simulink model "projectmodel"  (R2016a)
settings: Solver=ode23tb  StartTime=0.0  StopTime=20  MaxStep=1e-3  RelTol=1e-3
values from neighbouring files (symbols this model uses):
  Supply_pr_Ps = 2.1e7    (= 21000000)    [data4_mfile.m]    (also in data8_mfile.m)
  Valve_eta = 0.989    [data4_mfile.m]    (also in data8_mfile.m = 0.99)
  Valve_omega = 40.5    [data4_mfile.m]    (also in data8_mfile.m = 38)
undefined symbols (not defined in the file or in its folder): Arm, Boom, Bucket, Cyl, Hose, Valve
libraries: mblibv1 x13, simulink x3, vrlib x2
settings Model: Creator=bangalor  LastModifiedBy=bangalor

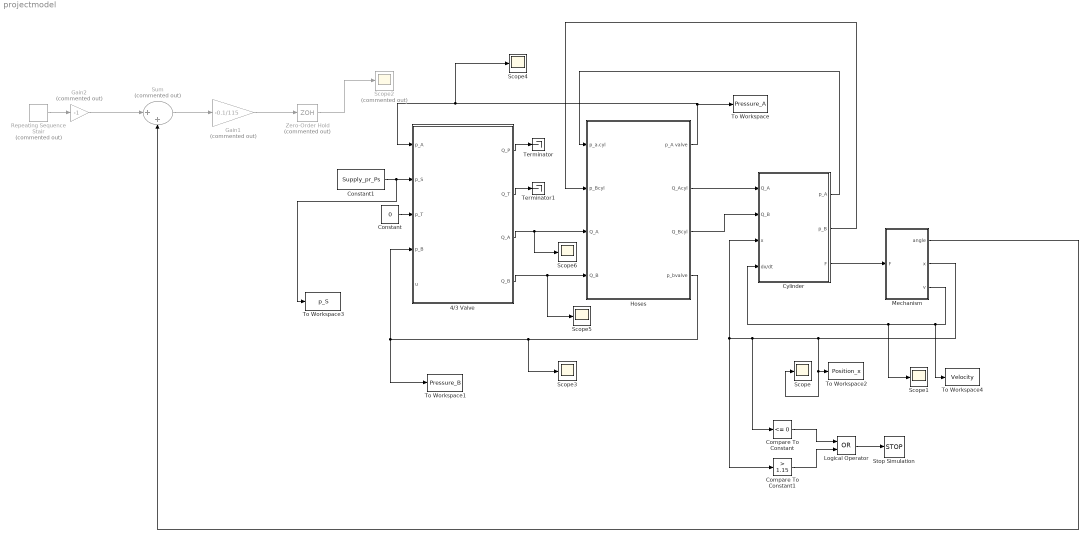
== system projectmodel ==
  4/3 Valve : Subsystem
  Compare To Constant : simulink/Logic and Bit Operations/Compare To Constant  relop=<=  const=0  OutDataTypeStr=boolean
  Compare To Constant1 : simulink/Logic and Bit Operations/Compare To Constant  relop=>  const=1.15  OutDataTypeStr=boolean
  Constant : Constant  Value=0
  Constant1 : Constant  Value=Supply_pr_Ps
  Cylinder : Subsystem
  Gain1 : Gain  Commented=on  Gain=-0.1/115
  Gain2 : Gain  Commented=on  Gain=-1
  Hoses : Subsystem
  Logical Operator : Logic  Operator=OR  AllPortsSameDT=off  OutDataTypeStr=boolean
  Mechanism : Subsystem
  Repeating Sequence Stair : simulink/Sources/Repeating Sequence Stair  Commented=on  OutValues=[50 72 94 115].'  tsamp=5  OutMin=[]  OutMax=[]  OutDataTypeStr=double  OutputDataTypeScalingMode=double  OutDataType=fixdt(0,8)  ConRadixGroup=Best Precision: Vector-wise  OutScaling=2^-12
  Scope{,1,3..6} (6 alike) : Scope
  Scope2 : Scope  Commented=on
  Stop Simulation : Stop
  Sum : Sum  Commented=on  Inputs=|++
  Terminator : Terminator
  Terminator1 : Terminator
  To Workspace : ToWorkspace  VariableName=Pressure_A  SampleTime=-1
  To Workspace1 : ToWorkspace  VariableName=Pressure_B  SampleTime=-1
  To Workspace2 : ToWorkspace  VariableName=Position_x  SampleTime=-1
  To Workspace3 : ToWorkspace  VariableName=p_S  SampleTime=-1
  To Workspace4 : ToWorkspace  VariableName=Velocity  SampleTime=-1
  Zero-Order Hold : ZeroOrderHold  Commented=on  SampleTime=50e-3
  wires:
  4/3 Valve/3(Q_A) -> Scope6/1, Hoses/3(Q_A)
  4/3 Valve/4(Q_B) -> Scope5/1, Hoses/4(Q_B)
  Mechanism/3(v) -> Cylinder/4(dx/dt), Scope1/1, To Workspace4/1
  Hoses/4(p_bvalve) -> Scope3/1, To Workspace1/1, 4/3 Valve/4(p_B)
  Hoses/1(p_A valve) -> Scope4/1, 4/3 Valve/1(p_A), To Workspace/1
  Hoses/2(Q_Acyl) -> Cylinder/1(Q_A)
  Hoses/3(Q_Bcyl) -> Cylinder/2(Q_B)
  Cylinder/1(p_A) -> Hoses/1(p_a.cyl)
  Cylinder/2(p_B) -> Hoses/2(p_Bcyl)
  4/3 Valve/1(Q_P) -> Terminator/1
  4/3 Valve/2(Q_T) -> Terminator1/1
  Constant/1 -> 4/3 Valve/3(p_T)
  Constant1/1 -> To Workspace3/1, 4/3 Valve/2(p_S)
  Cylinder/3(F) -> Mechanism/1(F)
  Sum/1 -> Gain1/1
  Gain1/1 -> Zero-Order Hold/1
  Mechanism/1(angle) -> Sum/2
  Repeating Sequence Stair/1 -> Gain2/1
  Zero-Order Hold/1 -> Scope2/1
  Gain2/1 -> Sum/1
  Mechanism/2(x) -> Scope/1, To Workspace2/1, Compare To Constant/1, Compare To Constant1/1, Cylinder/3(x)
  Compare To Constant/1 -> Logical Operator/1
  Compare To Constant1/1 -> Logical Operator/2
  Logical Operator/1 -> Stop Simulation/1

== system projectmodel/4//3 Valve ==
  p_A : Inport
  p_S : Inport  Port=2
  p_T : Inport  Port=3
  p_B : Inport  Port=4
  u : Inport  Port=5
  Flow paths : Subsystem
  From Workspace : FromWorkspace  VariableName=U_signal  SampleTime=1.0000e-03
  Relative openings : Subsystem
  Scope6 : Scope
  Valve Dynamics : Subsystem
  Q_P : Outport
  Q_T : Outport  Port=2
  Q_A : Outport  Port=3
  Q_B : Outport  Port=4
  wires:
  Valve Dynamics/1(x) -> Scope6/1, Relative openings/1(x)
  Relative openings/1(av_AT) -> Flow paths/5(av_AT)
  Flow paths/4(Q_B) -> Q_B/1
  Flow paths/3(Q_T) -> Q_T/1
  Flow paths/2(Q_P) -> Q_P/1
  Flow paths/1(Q_A) -> Q_A/1
  p_T/1 -> Flow paths/4(p_T)
  p_S/1 -> Flow paths/3(p_S)
  p_B/1 -> Flow paths/2(p_B)
  p_A/1 -> Flow paths/1(p_A)
  Relative openings/2(av_BT) -> Flow paths/6(av_BT)
  Relative openings/3(av_PB) -> Flow paths/7(av_PB)
  Relative openings/4(av_PA) -> Flow paths/8(av_PA)
  From Workspace/1 -> Valve Dynamics/1(u)

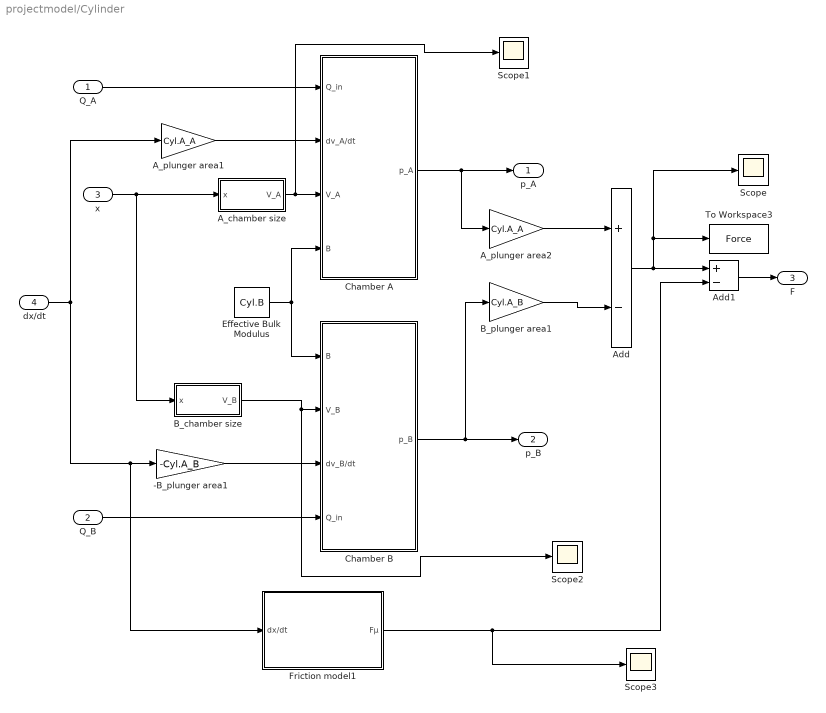
== system projectmodel/Cylinder ==
  Q_A : Inport
  Q_B : Inport  Port=2
  x : Inport  Port=3
  dx/dt : Inport  Port=4
  -B_plunger area1 : Gain  Gain=-Cyl.A_B
  A_chamber size : Subsystem
  A_plunger area1 : Gain  Gain=Cyl.A_A
  A_plunger area2 : Gain  Gain=Cyl.A_A
  Add : Sum  Inputs=+-
  Add1 : Sum  Inputs=+-
  B_chamber size : Subsystem
  B_plunger area1 : Gain  Gain=Cyl.A_B
  Chamber A : Subsystem  mask(Hydraulic){pinitial=Cyl.pa_init}
      mask prompts: pinitial "Initial pressure [Pa] :"
      mask help: Lumped fluid volume. Pressure is limited greater or equal to zero by saturation block corresponding to a rough model of cavitation.
      mask Help: eval('hydlibdoc(''vol_cav_doc'')')
  Chamber B : Subsystem  mask(Hydraulic){pinitial=Cyl.pb_init}
      mask prompts: pinitial "Initial pressure [Pa] :"
      mask help: Lumped fluid volume. Pressure is limited greater or equal to zero by saturation block corresponding to a rough model of cavitation.
      mask Help: eval('hydlibdoc(''vol_cav_doc'')')
  Effective Bulk Modulus : Constant  Value=Cyl.B
  Friction model1 : Subsystem
  Scope{,1..3} (4 alike) : Scope
  To Workspace3 : ToWorkspace  VariableName=Force  SampleTime=-1
  p_A : Outport
  p_B : Outport  Port=2
  F : Outport  Port=3
  wires:
  A_plunger area1/1 -> Chamber A/2(" dv_A/dt")
  dx/dt/1 -> A_plunger area1/1, Friction model1/1(dx/dt), -B_plunger area1/1
  Effective Bulk Modulus/1 -> Chamber A/4(" B"), Chamber B/1(B)
  x/1 -> B_chamber size/1(x), A_chamber size/1(x)
  -B_plunger area1/1 -> Chamber B/3(dv_B/dt)
  A_chamber size/1(V_A) -> Scope1/1, Chamber A/3(" V_A")
  Friction model1/1(Fµ) -> Add1/2, Scope3/1
  Q_A/1 -> Chamber A/1(Q_in)
  Chamber A/1(p_A) -> p_A/1, A_plunger area2/1
  Chamber B/1(p_B) -> p_B/1, B_plunger area1/1
  A_plunger area2/1 -> Add/1
  B_plunger area1/1 -> Add/2
  Add/1 -> Add1/1, To Workspace3/1, Scope/1
  B_chamber size/1(V_B) -> Scope2/1, Chamber B/2(V_B)
  Q_B/1 -> Chamber B/4(Q_in)
  Add1/1 -> F/1

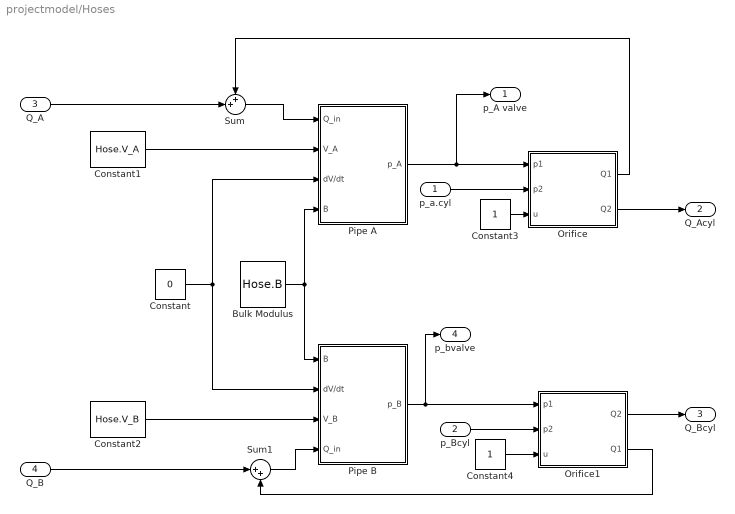
== system projectmodel/Hoses ==
  p_a.cyl : Inport
  p_Bcyl : Inport  Port=2
  Q_A : Inport  Port=3
  Q_B : Inport  Port=4
  Bulk Modulus : Constant  Value=Hose.B
  Constant : Constant  Value=0
  Constant1 : Constant  Value=Hose.V_A
  Constant2 : Constant  Value=Hose.V_B
  Constant3 : Constant
  Constant4 : Constant
  Orifice : Subsystem  mask(Hydraulic){QN=Hose.QN, dpN=Hose.dpN, ptr=Hose.ptr}
      mask prompts: QN "Nominal Flow [m^3/s] :"; dpN "Nominal Pressure Difference [Pa] :"; ptr "Transition Pressure [Pa] :"
      mask help:
      | Implements numerically robust turbulent flow
      | equation. Polynomial flow equation is used
      | when abs(dp) < Transition Pressure.
      mask init:
      | K = QN/(sqrt(dpN));
      mask Help: eval('hydlibdoc(''orificedoc'')')
  Orifice1 : Subsystem  mask(Hydraulic){QN=Hose.QN, dpN=Hose.dpN, ptr=Hose.ptr}
      mask prompts: QN "Nominal Flow [m^3/s] :"; dpN "Nominal Pressure Difference [Pa] :"; ptr "Transition Pressure [Pa] :"
      mask help:
      | Implements numerically robust turbulent flow
      | equation. Polynomial flow equation is used
      | when abs(dp) < Transition Pressure.
      mask init:
      | K = QN/(sqrt(dpN));
      mask Help: eval('hydlibdoc(''orificedoc'')')
  Pipe A : Subsystem  mask(Hydraulic){pinitial=Hose.pa_init}
      mask prompts: pinitial "Initial pressure [Pa] :"
      mask help: Lumped fluid volume. Pressure is limited greater or equal to zero by saturation block corresponding to a rough model of cavitation.
      mask Help: eval('hydlibdoc(''vol_cav_doc'')')
  Pipe B : Subsystem  mask(Hydraulic){pinitial=Hose.pb_init}
      mask prompts: pinitial "Initial pressure [Pa] :"
      mask help: Lumped fluid volume. Pressure is limited greater or equal to zero by saturation block corresponding to a rough model of cavitation.
      mask Help: eval('hydlibdoc(''vol_cav_doc'')')
  Sum : Sum  Inputs=++|
  Sum1 : Sum  Inputs=|++
  p_A valve : Outport
  Q_Acyl : Outport  Port=2
  Q_Bcyl : Outport  Port=3
  p_bvalve : Outport  Port=4
  wires:
  Q_B/1 -> Sum1/1
  Constant4/1 -> Orifice1/3(u)
  Constant2/1 -> Pipe B/3(V_B)
  Pipe A/1(p_A) -> p_A valve/1, Orifice/1(p1)
  p_a.cyl/1 -> Orifice/2(p2)
  Orifice/1(Q1) -> Sum/1
  Orifice/2(Q2) -> Q_Acyl/1
  Q_A/1 -> Sum/2
  Sum/1 -> Pipe A/1(Q_in)
  Pipe B/1(p_B) -> p_bvalve/1, Orifice1/1(p1)
  Orifice1/2(Q1) -> Sum1/2
  Sum1/1 -> Pipe B/4(" Q_in")
  Orifice1/1(Q2) -> Q_Bcyl/1
  Bulk Modulus/1 -> Pipe A/4(" B"), Pipe B/1(B)
  Constant/1 -> Pipe A/3(" dV/dt"), Pipe B/2(" dV/dt")
  Constant1/1 -> Pipe A/2(" V_A")
  Constant3/1 -> Orifice/3(u)
  p_Bcyl/1 -> Orifice1/2(p2)

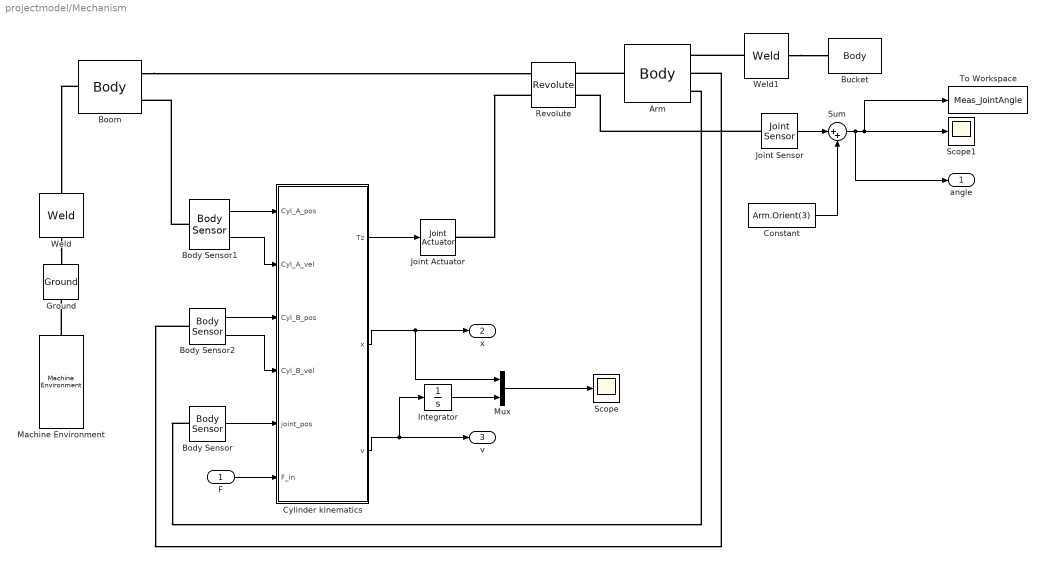
== system projectmodel/Mechanism ==
  F : Inport
  Arm : mblibv1/Bodies/Body  LConnTagsString=CS1  RConnTagsString=CS3|CS2|CS4  UpdateFromCAD=off  DialogClass=MechanicalBodyBlock  Mass=Arm.Mass  MassUnits=kg  InertiaUnits=kg*m^2  Inertia=Arm.Inertia  Shape=Cylinder  ShapeDims=[1 1]  ShapeUnits=m  ShapeUse=false  Density=1  DensityUnits=kg/m^3  DensityUse=false  GraphicsMode=MACHINE_DEFAULT  BodyColorSelMode=MACHINE_DEFAULT  BodyColor=[1 0 0]  AttachedToCS=CG  CG=Left$CG$Arm.CG$CS1$CS1$m$[0 0 0]$Euler X-Y-Z$deg$CS1$false$none  WorkingFrames=Left$CS1$[0 0 0]$Adjoining$Adjoining$m$Arm.Orient$Euler X-Y-Z$deg$Adjoining$true$none#Right$CS3$Arm.BucketJoint$CS1$CS1$m$[0 0 0]$Euler X-Y-Z$deg$CS1$true$none#Right$CS2$Arm.CylJoint$CS1$CS1$m$[0 0 0]$Euler X-Y-Z$deg$CS1$true$none#Right$CS4$[0 0 0]$CS1$CS1$m$[0 0 0]$Euler X-Y-Z$deg$CS1$true$none  CGPos=Arm.CG  CGRot=[0 0 0]  CS0Pos=[]  CS0Rot=[]  CS1Pos=[0 0 0]  CS1Rot=Arm.Orient  CS2Pos=Arm.CylJoint  CS2Rot=[0 0 0]  CS3Pos=Arm.BucketJoint  CS3Rot=[0 0 0]  CS4Pos=[0 0 0]  CS4Rot=[0 0 0]  CS5Pos=[]  CS5Rot=[]  CS6Pos=[]  CS6Rot=[]  CS7Pos=[]  CS7Rot=[]  CS8Pos=[]  CS8Rot=[]  CS9Pos=[]  CS9Rot=[]  CS10Pos=[]  CS10Rot=[]  CS11Pos=[]  CS11Rot=[]  CS12Pos=[]  CS12Rot=[]  CS13Pos=[]  CS13Rot=[]  CS14Pos=[]  CS14Rot=[]  CS15Pos=[]  CS15Rot=[]  CS16Pos=[]  CS16Rot=[]  CS17Pos=[]  CS17Rot=[]  CS18Pos=[]  CS18Rot=[]  CS19Pos=[]  CS19Rot=[]  CS20Pos=[]  CS20Rot=[]
  Body Sensor : mblibv1/Sensors &  Actuators/Body Sensor  UpdateFromCAD=off  PhysicalDomain=Mechanical  PortType=blob  Muxed=off  Pose=off  Angle=on  AngleUnits=deg  ArcVelocity=off  ArcVelocityUnits=deg/s  ArcAcceleration=off  ArcAccelerationUnits=deg/s^2  CoordPosition=on  CoordPositionUnits=m  Velocity=off  VelocityUnits=m/s  Acceleration=off  AccelerationUnits=m/s^2  Quaternion=on  QuaternionDT=off  QuaternionDDT=off  QuaternionUnits=off  OutputVector=[1]  ActiveIO=on  Width=3  DialogClass=MechanicalSensorBlock  ReferenceFrame=Absolute (World)
  Body Sensor1 : mblibv1/Sensors &  Actuators/Body Sensor  UpdateFromCAD=off  PhysicalDomain=Mechanical  PortType=blob  Muxed=off  Pose=off  Angle=on  AngleUnits=deg  ArcVelocity=off  ArcVelocityUnits=deg/s  ArcAcceleration=off  ArcAccelerationUnits=deg/s^2  CoordPosition=on  CoordPositionUnits=m  Velocity=on  VelocityUnits=m/s  Acceleration=off  AccelerationUnits=m/s^2  Quaternion=on  QuaternionDT=off  QuaternionDDT=off  QuaternionUnits=off  OutputVector=[1]  ActiveIO=on  Width=6  DialogClass=MechanicalSensorBlock  ReferenceFrame=Absolute (World)
  Body Sensor2 : mblibv1/Sensors &  Actuators/Body Sensor  UpdateFromCAD=off  PhysicalDomain=Mechanical  PortType=blob  Muxed=off  Pose=off  Angle=on  AngleUnits=deg  ArcVelocity=off  ArcVelocityUnits=deg/s  ArcAcceleration=off  ArcAccelerationUnits=deg/s^2  CoordPosition=on  CoordPositionUnits=m  Velocity=on  VelocityUnits=m/s  Acceleration=off  AccelerationUnits=m/s^2  Quaternion=on  QuaternionDT=off  QuaternionDDT=off  QuaternionUnits=off  OutputVector=[1]  ActiveIO=on  Width=6  DialogClass=MechanicalSensorBlock  ReferenceFrame=Absolute (World)
  Boom : mblibv1/Bodies/Body  LConnTagsString=CS1  RConnTagsString=CS2|CS3  UpdateFromCAD=off  DialogClass=MechanicalBodyBlock  Mass=Boom.Mass  MassUnits=kg  InertiaUnits=kg*m^2  Inertia=Boom.Inert  Shape=Cylinder  ShapeDims=[1 1]  ShapeUnits=m  ShapeUse=false  Density=1  DensityUnits=kg/m^3  DensityUse=false  GraphicsMode=MACHINE_DEFAULT  BodyColorSelMode=MACHINE_DEFAULT  BodyColor=[1 0 0]  AttachedToCS=CG  CG=Left$CG$[0 0 0]$CS1$CS1$m$[0 0 0]$Euler X-Y-Z$deg$CS1$false$none  WorkingFrames=Left$CS1$[0 0 0]$Adjoining$Adjoining$m$[0 0 0]$Euler X-Y-Z$deg$Adjoining$true$none#Right$CS2$Boom.ArmJoint$CS1$CS1$m$[0 0 0]$Euler X-Y-Z$deg$CS1$true$none#Right$CS3$Boom.CylJoint$CS1$CS1$m$[0 0 0]$Euler X-Y-Z$deg$CS1$true$none  CGPos=[0 0 0]  CGRot=[0 0 0]  CS0Pos=[]  CS0Rot=[]  CS1Pos=[0 0 0]  CS1Rot=[0 0 0]  CS2Pos=Boom.ArmJoint  CS2Rot=[0 0 0]  CS3Pos=Boom.CylJoint  CS3Rot=[0 0 0]  CS4Pos=[]  CS4Rot=[]  CS5Pos=[]  CS5Rot=[]  CS6Pos=[]  CS6Rot=[]  CS7Pos=[]  CS7Rot=[]  CS8Pos=[]  CS8Rot=[]  CS9Pos=[]  CS9Rot=[]  CS10Pos=[]  CS10Rot=[]  CS11Pos=[]  CS11Rot=[]  CS12Pos=[]  CS12Rot=[]  CS13Pos=[]  CS13Rot=[]  CS14Pos=[]  CS14Rot=[]  CS15Pos=[]  CS15Rot=[]  CS16Pos=[]  CS16Rot=[]  CS17Pos=[]  CS17Rot=[]  CS18Pos=[]  CS18Rot=[]  CS19Pos=[]  CS19Rot=[]  CS20Pos=[]  CS20Rot=[]
  Bucket : mblibv1/Bodies/Body  LConnTagsString=CS1  UpdateFromCAD=off  DialogClass=MechanicalBodyBlock  Mass=Bucket.Mass  MassUnits=kg  InertiaUnits=kg*m^2  Inertia=Bucket.Interia  Shape=Cylinder  ShapeDims=[1 1]  ShapeUnits=m  ShapeUse=false  Density=1  DensityUnits=kg/m^3  DensityUse=false  GraphicsMode=MACHINE_DEFAULT  BodyColorSelMode=MACHINE_DEFAULT  BodyColor=[1 0 0]  AttachedToCS=CG  CG=Left$CG$Bucket.CG$CS1$CS1$m$[0 0 0]$Euler X-Y-Z$deg$CS1$false$none  WorkingFrames=Left$CS1$[0 0 0]$Adjoining$Adjoining$m$[0 0 0]$Euler X-Y-Z$deg$Adjoining$true$none  CGPos=Bucket.CG  CGRot=[0 0 0]  CS0Pos=[]  CS0Rot=[]  CS1Pos=[0 0 0]  CS1Rot=[0 0 0]  CS2Pos=[]  CS2Rot=[]  CS3Pos=[]  CS3Rot=[]  CS4Pos=[]  CS4Rot=[]  CS5Pos=[]  CS5Rot=[]  CS6Pos=[]  CS6Rot=[]  CS7Pos=[]  CS7Rot=[]  CS8Pos=[]  CS8Rot=[]  CS9Pos=[]  CS9Rot=[]  CS10Pos=[]  CS10Rot=[]  CS11Pos=[]  CS11Rot=[]  CS12Pos=[]  CS12Rot=[]  CS13Pos=[]  CS13Rot=[]  CS14Pos=[]  CS14Rot=[]  CS15Pos=[]  CS15Rot=[]  CS16Pos=[]  CS16Rot=[]  CS17Pos=[]  CS17Rot=[]  CS18Pos=[]  CS18Rot=[]  CS19Pos=[]  CS19Rot=[]  CS20Pos=[]  CS20Rot=[]
  Constant : Constant  Value=Arm.Orient(3)
  Cylinder kinematics : Subsystem
  Ground : mblibv1/Bodies/Ground  UpdateFromCAD=off  LeftPortType=env  RightPortType=workingframe  PhysicalDomain=Mechanical  DialogClass=GroundBlock  CoordPosition=[0 0 0]  CoordPositionUnits=m  StateVectorMgrId=0  MachineId=[1 0]  ShowEnvPort=on  ParameterChecksum=[1109649174, 3994819602, 1548314123, 2838236953]  TopologyChecksum=[2762165800, 3161043779, 663838886, 4152578307]
  Integrator : Integrator
  Joint Actuator : mblibv1/Sensors &  Actuators/Joint Actuator  UpdateFromCAD=off  PhysicalDomain=Mechanical  PortType=blob  ActuationStyle=Force  AngleUnits=deg  ArcVelocityUnits=deg/s  ArcAccelerationUnits=deg/s^2  CoordPositionUnits=m  VelocityUnits=m/s  AccelerationUnits=m/s^2  ForceUnits=N  TorqueUnits=N-m  ActiveIO=on  Width=1  DialogClass=MechanicalActuatorBlock  Primitive=R1  ReferenceFrame=Absolute (World)
  Joint Sensor : mblibv1/Sensors &  Actuators/Joint Sensor  UpdateFromCAD=off  PhysicalDomain=Mechanical  PortType=blob  Muxed=on  Pose=off  Angle=on  AngleUnits=deg  ArcVelocity=off  ArcVelocityUnits=deg/s  ArcAcceleration=off  ArcAccelerationUnits=deg/s^2  CoordPosition=on  CoordPositionUnits=m  Velocity=off  VelocityUnits=m/s  Acceleration=off  AccelerationUnits=m/s^2  Quaternion=on  QuaternionDT=off  QuaternionDDT=off  QuaternionUnits=off  OutputVector=[1]  ActiveIO=on  Width=1  DialogClass=MechanicalSensorBlock  Primitive=R1  Force=off  ForceUnits=N  Torque=off  TorqueUnits=N-m  ReferenceFrame=Absolute (World)  ReactionSensedSide=Base  ReactionReferenceFrame=Absolute (World)  ReactionForce=off  ReactionForceUnits=N  ReactionMoment=off  ReactionMomentUnits=N-m
  Machine Environment : mblibv1/Bodies/Machine Environment  PortType=env  PhysicalDomain=Mechanical  DialogTemplateClass=MECH.MachineEnvironment  SyncWhenCopied=off  Gravity=[0 -9.81 0]  GravityUnits=m/s^2  GravityAsSignal=off  Dimensionality=Auto-detect  AnalysisType=Forward dynamics  LinearAssemblyTolerance=1e-3  LinearAssemblyToleranceUnits=m  AngularAssemblyTolerance=1e-3  AngularAssemblyToleranceUnits=rad  ConstraintSolverType=Stabilizing  ConstraintRelTolerance=1e-4  ConstraintAbsTolerance=1e-4  UseRobustSingularityHandling=off  RedundancyAnalysisToleranceType=Automatically select tolerance  RedundancyAnalysisTolerance=1e-14  StatePerturbationType=Fixed  PerturbationSize=1e-5  VisualizeMachine=on  BodyVisualizationType=Use model default body geometries  BodyColorSelMode=Use model default  DefaultBodyColor=[1 0 0]
  Mux : Mux  Inputs=2
  Revolute : mblibv1/Joints/Revolute  LConnTagsString=__newl0|SA1  RConnTagsString=__newr0|SA1  UpdateFromCAD=off  NumSAPorts=2  CutJoint=off  MarkAsCut=off  Primitives=prismatic  PrimitiveProps=R1$World$[0 0 1]$revolute  DialogClass=JointBlock  R1Axis=[0 0 1]
  Scope : Scope
  Scope1 : Scope
  Sum : Sum  Inputs=|++
  To Workspace : ToWorkspace  VariableName=Meas_JointAngle  SampleTime=-1
  Weld : mblibv1/Joints/Weld  LConnTagsString=__newl0  RConnTagsString=__newr0  UpdateFromCAD=off  NumSAPorts=0  CutJoint=off  MarkAsCut=off  Primitives=weld  PrimitiveProps=W$WORLD$[0 0 0]$weld  DialogClass=JointBlock  WAxis=[0 0 0]
  Weld1 : mblibv1/Joints/Weld  LConnTagsString=__newl0  RConnTagsString=__newr0  UpdateFromCAD=off  NumSAPorts=0  CutJoint=off  MarkAsCut=off  Primitives=weld  PrimitiveProps=W$WORLD$[0 0 0]$weld  DialogClass=JointBlock  WAxis=[0 0 0]
  angle : Outport
  x : Outport  Port=2
  v : Outport  Port=3
  wires:
  Cylinder kinematics/1(Tz) -> Joint Actuator/1
  Joint Sensor/1 -> Sum/1
  F/1 -> Cylinder kinematics/6(F_in)
  Body Sensor/1 -> Cylinder kinematics/5(joint_pos)
  Cylinder kinematics/3(v) -> v/1, Integrator/1
  Cylinder kinematics/2(x) -> x/1, Mux/1
  Integrator/1 -> Mux/2
  Mux/1 -> Scope/1
  Body Sensor2/1 -> Cylinder kinematics/3(Cyl_B_pos)
  Body Sensor1/1 -> Cylinder kinematics/1(Cyl_A_pos)
  Body Sensor1/2 -> Cylinder kinematics/2(Cyl_A_vel)
  Body Sensor2/2 -> Cylinder kinematics/4(Cyl_B_vel)
  Constant/1 -> Sum/2
  Sum/1 -> angle/1, Scope1/1, To Workspace/1
  connections:
  Body Sensor1/LConn1 -- Boom/RConn2
  Weld/LConn1 -- Ground/RConn1
  Boom/LConn1 -- Weld/RConn1
  Arm/LConn1 -- Revolute/RConn1
  Machine Environment/RConn1 -- Ground/LConn1
  Weld1/LConn1 -- Arm/RConn1
  Weld1/RConn1 -- Bucket/LConn1
  Revolute/LConn2 -- Joint Actuator/RConn1
  Body Sensor2/LConn1 -- Arm/RConn2
  Body Sensor/LConn1 -- Arm/RConn3
  Boom/RConn1 -- Revolute/LConn1
  Joint Sensor/LConn1 -- Revolute/RConn2

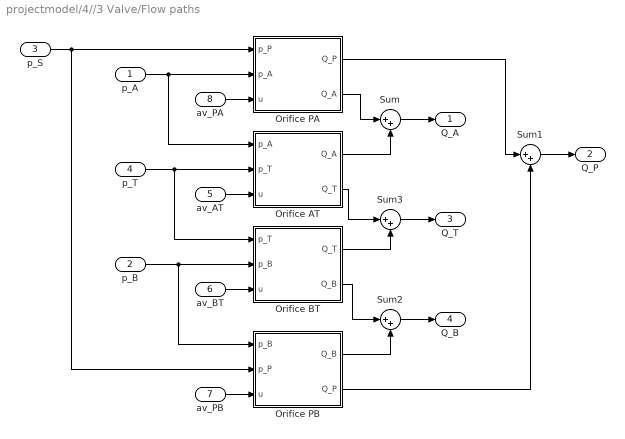
== system projectmodel/4//3 Valve/Flow paths ==
  p_A : Inport
  p_B : Inport  Port=2
  p_S : Inport  Port=3
  p_T : Inport  Port=4
  av_AT : Inport  Port=5
  av_BT : Inport  Port=6
  av_PB : Inport  Port=7
  av_PA : Inport  Port=8
  Orifice AT : Subsystem  mask(Hydraulic){QN=Valve.QN.AT, dpN=Valve.dpN, ptr=Valve.ptr}
      mask prompts: QN "Nominal Flow [m^3/s] :"; dpN "Nominal Pressure Difference [Pa] :"; ptr "Transition Pressure [Pa] :"
      mask help:
      | Implements numerically robust turbulent flow
      | equation. Polynomial flow equation is used
      | when abs(dp) < Transition Pressure.
      mask init:
      | K = QN/(sqrt(dpN));
      mask Help: eval('hydlibdoc(''orificedoc'')')
  Orifice BT : Subsystem  mask(Hydraulic){QN=Valve.QN.BT, dpN=Valve.dpN, ptr=Valve.ptr}
      mask prompts: QN "Nominal Flow [m^3/s] :"; dpN "Nominal Pressure Difference [Pa] :"; ptr "Transition Pressure [Pa] :"
      mask help:
      | Implements numerically robust turbulent flow
      | equation. Polynomial flow equation is used
      | when abs(dp) < Transition Pressure.
      mask init:
      | K = QN/(sqrt(dpN));
      mask Help: eval('hydlibdoc(''orificedoc'')')
  Orifice PA : Subsystem  mask(Hydraulic){QN=Valve.QN.PA, dpN=Valve.dpN, ptr=Valve.ptr}
      mask prompts: QN "Nominal Flow [m^3/s] :"; dpN "Nominal Pressure Difference [Pa] :"; ptr "Transition Pressure [Pa] :"
      mask help:
      | Implements numerically robust turbulent flow
      | equation. Polynomial flow equation is used
      | when abs(dp) < Transition Pressure.
      mask init:
      | K = QN/(sqrt(dpN));
      mask Help: eval('hydlibdoc(''orificedoc'')')
  Orifice PB : Subsystem  mask(Hydraulic){QN=Valve.QN.PB, dpN=Valve.dpN, ptr=Valve.ptr}
      mask prompts: QN "Nominal Flow [m^3/s] :"; dpN "Nominal Pressure Difference [Pa] :"; ptr "Transition Pressure [Pa] :"
      mask help:
      | Implements numerically robust turbulent flow
      | equation. Polynomial flow equation is used
      | when abs(dp) < Transition Pressure.
      mask init:
      | K = QN/(sqrt(dpN));
      mask Help: eval('hydlibdoc(''orificedoc'')')
  Sum{,1..3} (4 alike) : Sum  Inputs=|++
  Q_A : Outport
  Q_P : Outport  Port=2
  Q_T : Outport  Port=3
  Q_B : Outport  Port=4
  wires:
  p_A/1 -> Orifice AT/1(p_A), Orifice PA/2(p_A)
  p_T/1 -> Orifice BT/1(p_T), Orifice AT/2(p_T)
  av_BT/1 -> Orifice BT/3(u)
  av_PA/1 -> Orifice PA/3(u)
  p_B/1 -> Orifice PB/1(p_B), Orifice BT/2(p_B)
  av_PB/1 -> Orifice PB/3(u)
  p_S/1 -> Orifice PB/2(p_P), Orifice PA/1(p_P)
  av_AT/1 -> Orifice AT/3(u)
  Orifice PA/2(Q_A) -> Sum/1
  Orifice AT/1(Q_A) -> Sum/2
  Orifice AT/2(Q_T) -> Sum3/1
  Orifice BT/1(Q_T) -> Sum3/2
  Orifice BT/2(Q_B) -> Sum2/1
  Orifice PB/1(Q_B) -> Sum2/2
  Orifice PA/1(Q_P) -> Sum1/1
  Orifice PB/2(Q_P) -> Sum1/2
  Sum/1 -> Q_A/1
  Sum1/1 -> Q_P/1
  Sum3/1 -> Q_T/1
  Sum2/1 -> Q_B/1

== system projectmodel/4//3 Valve/Relative openings ==
  x : Inport
  Lookup Table AT : Lookup_n-D  NumberOfTableDimensions=1  BreakpointsForDimension1=Valve.lookupspoolAT  Table=Valve.lookupopenAT  InternalRulePriority=Speed  RndMeth=Simplest  InputSameDT=on
  Lookup Table BT : Lookup_n-D  NumberOfTableDimensions=1  BreakpointsForDimension1=Valve.lookupspoolBT  Table=Valve.lookupopenBT  InternalRulePriority=Speed  RndMeth=Simplest  InputSameDT=on
  Lookup Table PA : Lookup_n-D  NumberOfTableDimensions=1  BreakpointsForDimension1=Valve.lookupspoolPA  Table=Valve.lookupopenPA  InternalRulePriority=Speed  RndMeth=Simplest  InputSameDT=on
  Lookup Table PB : Lookup_n-D  NumberOfTableDimensions=1  BreakpointsForDimension1=Valve.lookupspoolPB  Table=Valve.lookupopenPB  InternalRulePriority=Speed  RndMeth=Simplest  InputSameDT=on
  av_AT : Outport
  av_BT : Outport  Port=2
  av_PB : Outport  Port=3
  av_PA : Outport  Port=4
  wires:
  x/1 -> Lookup Table AT/1, Lookup Table PB/1, Lookup Table BT/1, Lookup Table PA/1
  Lookup Table AT/1 -> av_AT/1
  Lookup Table PA/1 -> av_PA/1
  Lookup Table BT/1 -> av_BT/1
  Lookup Table PB/1 -> av_PB/1

== system projectmodel/4//3 Valve/Valve Dynamics ==
  u : Inport
  Saturation1 : Saturate  UpperLimit=1  LowerLimit=-1
  Scope : Scope
  To Workspace : ToWorkspace  VariableName=x_spool  SampleTime=-1
  Transfer Fcn1 : TransferFcn  Numerator=[(Valve_omega)^2]  Denominator=[1 2*Valve_eta*Valve_omega (Valve_omega)^2]
  Transport Delay1 : TransportDelay  DelayTime=Valve.secondorder_delay
  x : Outport
  wires:
  Transfer Fcn1/1 -> Scope/1, Saturation1/1
  u/1 -> Transport Delay1/1
  Saturation1/1 -> To Workspace/1, x/1
  Transport Delay1/1 -> Transfer Fcn1/1

== system projectmodel/Cylinder/A_chamber size ==
  x : Inport
  A_Dead Vol : Constant  Value=Cyl.V0A
  A_plunger area : Gain  Gain=Cyl.A_A
  Add1 : Sum
  V_A : Outport
  wires:
  A_Dead Vol/1 -> Add1/2
  A_plunger area/1 -> Add1/1
  x/1 -> A_plunger area/1
  Add1/1 -> V_A/1

== system projectmodel/Cylinder/B_chamber size ==
  x : Inport
  Add2 : Sum  Inputs=-+
  Add4 : Sum
  B_Dead Vol : Constant  Value=Cyl.V0B
  B_plunger area : Gain  Gain=Cyl.A_B
  Cyl_stroke : Constant  Value=Cyl.xmax
  V_B : Outport
  wires:
  Add4/1 -> V_B/1
  B_Dead Vol/1 -> Add4/2
  B_plunger area/1 -> Add4/1
  Add2/1 -> B_plunger area/1
  x/1 -> Add2/1
  Cyl_stroke/1 -> Add2/2

== system projectmodel/Cylinder/Chamber A ==
  Q_in : Inport
  " dv_A/dt" : Inport  Port=2
  " V_A" : Inport  Port=3
  " B" : Inport  Port=4
  Integrator : Integrator  InitialCondition=pinitial  AbsoluteTolerance=10
  Product : Product  Inputs=*/*  SaturateOnIntegerOverflow=on  InputSameDT=on  OutDataTypeStr=Inherit: Same as first input
  Saturation : Saturate  UpperLimit=inf  LowerLimit=0
  Sum : Sum  Inputs=+-  SaturateOnIntegerOverflow=on  InputSameDT=on  OutDataTypeStr=Inherit: Same as first input
  p_A : Outport
  wires:
  Sum/1 -> Product/1
  Q_in/1 -> Sum/1
  " B"/1 -> Product/3
  Saturation/1 -> p_A/1
  Integrator/1 -> Saturation/1
  Product/1 -> Integrator/1
  " dv_A/dt"/1 -> Sum/2
  " V_A"/1 -> Product/2

== system projectmodel/Cylinder/Chamber B ==
  B : Inport
  V_B : Inport  Port=2
  dv_B/dt : Inport  Port=3
  Q_in : Inport  Port=4
  Integrator : Integrator  InitialCondition=pinitial  AbsoluteTolerance=10
  Product : Product  Inputs=*/*  SaturateOnIntegerOverflow=on  InputSameDT=on  OutDataTypeStr=Inherit: Same as first input
  Saturation : Saturate  UpperLimit=inf  LowerLimit=0
  Sum : Sum  Inputs=+-  SaturateOnIntegerOverflow=on  InputSameDT=on  OutDataTypeStr=Inherit: Same as first input
  p_B : Outport
  wires:
  Product/1 -> Integrator/1
  Integrator/1 -> Saturation/1
  Saturation/1 -> p_B/1
  B/1 -> Product/3
  Q_in/1 -> Sum/1
  Sum/1 -> Product/1
  dv_B/dt/1 -> Sum/2
  V_B/1 -> Product/2

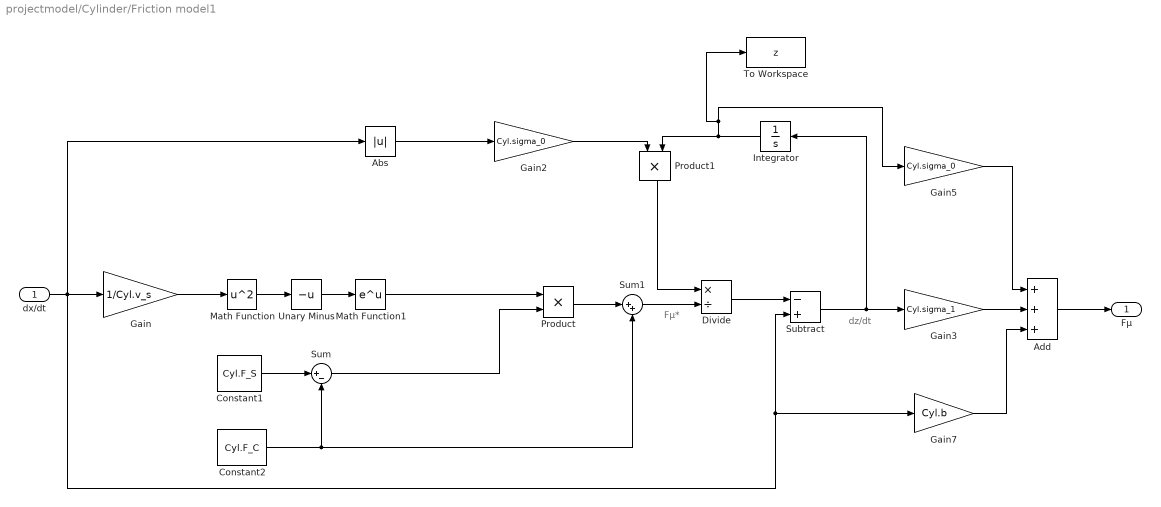
== system projectmodel/Cylinder/Friction model1 ==
  note: dz/dt
  note: Fµ*
  dx/dt : Inport
  Abs : Abs
  Add : Sum  Inputs=+++
  Constant1 : Constant  Value=Cyl.F_S
  Constant2 : Constant  Value=Cyl.F_C
  Divide : Product  Inputs=*/  SaturateOnIntegerOverflow=on  RndMeth=Zero
  Gain : Gain  Gain=1/Cyl.v_s
  Gain2 : Gain  Gain=Cyl.sigma_0
  Gain3 : Gain  Gain=Cyl.sigma_1
  Gain5 : Gain  Gain=Cyl.sigma_0
  Gain7 : Gain  Gain=Cyl.b
  Integrator : Integrator  AbsoluteTolerance=1e-12
  Math Function : Math  Operator=square  SaturateOnIntegerOverflow=on
  Math Function1 : Math  SaturateOnIntegerOverflow=on
  Product : Product
  Product1 : Product
  Subtract : Sum  Inputs=-+
  Sum : Sum  Inputs=|+-
  Sum1 : Sum  Inputs=|++
  To Workspace : ToWorkspace  VariableName=z  SampleTime=-1
  Unary Minus : UnaryMinus
  Fµ : Outport
  wires:
  Unary Minus/1 -> Math Function1/1
  Gain/1 -> Math Function/1
  dx/dt/1 -> Gain7/1, Subtract/2, Abs/1, Gain/1
  Abs/1 -> Gain2/1
  Gain2/1 -> Product1/1
  Subtract/1 -> Gain3/1, Integrator/1
  Math Function/1 -> Unary Minus/1
  Constant2/1 -> Sum1/2, Sum/2
  Math Function1/1 -> Product/1
  Sum/1 -> Product/2
  Constant1/1 -> Sum/1
  Product/1 -> Sum1/1
  Sum1/1 -> Divide/2
  Add/1 -> Fµ/1
  Gain3/1 -> Add/2
  Integrator/1 -> Product1/2, To Workspace/1, Gain5/1
  Product1/1 -> Divide/1
  Divide/1 -> Subtract/1
  Gain5/1 -> Add/1
  Gain7/1 -> Add/3

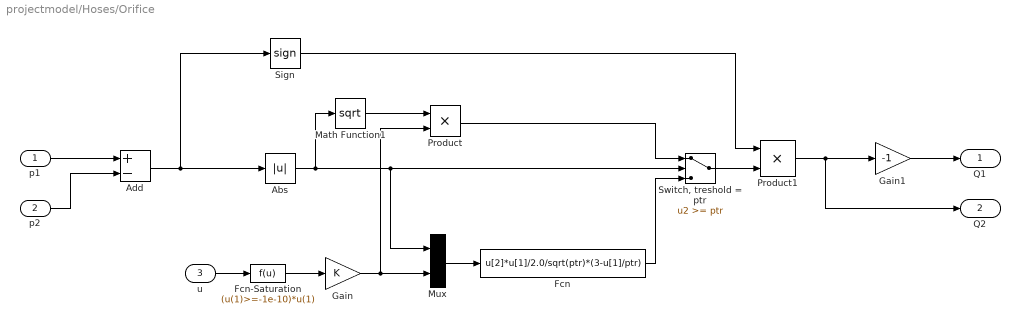
== system projectmodel/Hoses/Orifice ==
  p1 : Inport
  p2 : Inport  Port=2
  u : Inport  Port=3
  Abs : Abs  ZeroCross=off  SaturateOnIntegerOverflow=on
  Add : Sum  Inputs=+-
  Fcn : Fcn  Expr=u[2]*u[1]/2.0/sqrt(ptr)*(3-u[1]/ptr)
  Fcn-Saturation : Fcn  Expr=(u(1)>=-1e-10)*u(1)
  Gain : Gain  Gain=K  SaturateOnIntegerOverflow=on  OutDataTypeStr=Inherit: Same as input  ParamDataTypeStr=Inherit: Same as input
  Gain1 : Gain  Gain=-1  SaturateOnIntegerOverflow=on  OutDataTypeStr=Inherit: Same as input  ParamDataTypeStr=Inherit: Same as input
  Math Function1 : Math  Operator=sqrt  SaturateOnIntegerOverflow=on
  Mux : Mux  Inputs=2
  Product : Product  SaturateOnIntegerOverflow=on  InputSameDT=on  OutDataTypeStr=Inherit: Same as first input
  Product1 : Product  SaturateOnIntegerOverflow=on  InputSameDT=on  OutDataTypeStr=Inherit: Same as first input
  Sign : Signum  ZeroCross=off
  "Switch, treshold = ptr" : Switch  Threshold=ptr  ZeroCross=off  SaturateOnIntegerOverflow=on
  Q1 : Outport  InitialOutput=0
  Q2 : Outport  Port=2  InitialOutput=0
  wires:
  u/1 -> Fcn-Saturation/1
  Fcn/1 -> "Switch, treshold = ptr"/3
  Mux/1 -> Fcn/1
  Product/1 -> "Switch, treshold = ptr"/1
  Math Function1/1 -> Product/1
  Abs/1 -> "Switch, treshold = ptr"/2, Mux/1, Math Function1/1
  Fcn-Saturation/1 -> Gain/1
  Gain/1 -> Product/2, Mux/2
  "Switch, treshold = ptr"/1 -> Product1/2
  Sign/1 -> Product1/1
  p1/1 -> Add/1
  p2/1 -> Add/2
  Add/1 -> Abs/1, Sign/1
  Product1/1 -> Q2/1, Gain1/1
  Gain1/1 -> Q1/1

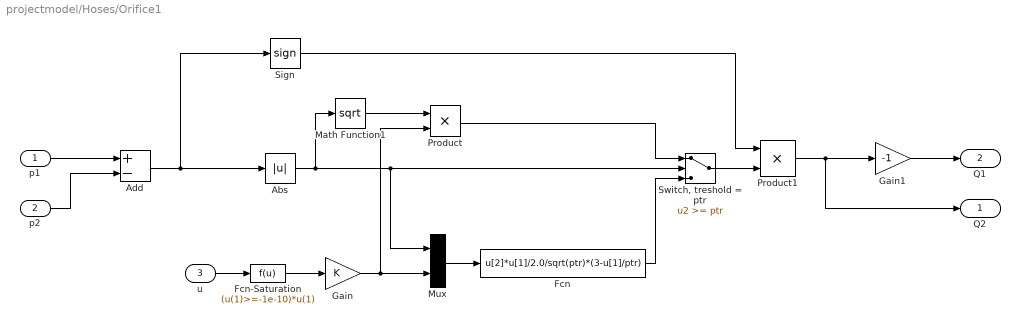
== system projectmodel/Hoses/Orifice1 ==
  p1 : Inport
  p2 : Inport  Port=2
  u : Inport  Port=3
  Abs : Abs  ZeroCross=off  SaturateOnIntegerOverflow=on
  Add : Sum  Inputs=+-
  Fcn : Fcn  Expr=u[2]*u[1]/2.0/sqrt(ptr)*(3-u[1]/ptr)
  Fcn-Saturation : Fcn  Expr=(u(1)>=-1e-10)*u(1)
  Gain : Gain  Gain=K  SaturateOnIntegerOverflow=on  OutDataTypeStr=Inherit: Same as input  ParamDataTypeStr=Inherit: Same as input
  Gain1 : Gain  Gain=-1  SaturateOnIntegerOverflow=on  OutDataTypeStr=Inherit: Same as input  ParamDataTypeStr=Inherit: Same as input
  Math Function1 : Math  Operator=sqrt  SaturateOnIntegerOverflow=on
  Mux : Mux  Inputs=2
  Product : Product  SaturateOnIntegerOverflow=on  InputSameDT=on  OutDataTypeStr=Inherit: Same as first input
  Product1 : Product  SaturateOnIntegerOverflow=on  InputSameDT=on  OutDataTypeStr=Inherit: Same as first input
  Sign : Signum  ZeroCross=off
  "Switch, treshold = ptr" : Switch  Threshold=ptr  ZeroCross=off  SaturateOnIntegerOverflow=on
  Q2 : Outport  InitialOutput=0
  Q1 : Outport  Port=2  InitialOutput=0
  wires:
  u/1 -> Fcn-Saturation/1
  Fcn/1 -> "Switch, treshold = ptr"/3
  Mux/1 -> Fcn/1
  Product/1 -> "Switch, treshold = ptr"/1
  Math Function1/1 -> Product/1
  Abs/1 -> "Switch, treshold = ptr"/2, Mux/1, Math Function1/1
  Fcn-Saturation/1 -> Gain/1
  Gain/1 -> Product/2, Mux/2
  "Switch, treshold = ptr"/1 -> Product1/2
  Sign/1 -> Product1/1
  p1/1 -> Add/1
  p2/1 -> Add/2
  Add/1 -> Abs/1, Sign/1
  Product1/1 -> Q2/1, Gain1/1
  Gain1/1 -> Q1/1

== system projectmodel/Hoses/Pipe A ==
  Q_in : Inport
  " V_A" : Inport  Port=2
  " dV/dt" : Inport  Port=3
  " B" : Inport  Port=4
  Integrator : Integrator  InitialCondition=pinitial  AbsoluteTolerance=10
  Product : Product  Inputs=*/*  SaturateOnIntegerOverflow=on  InputSameDT=on  OutDataTypeStr=Inherit: Same as first input
  Saturation : Saturate  UpperLimit=inf  LowerLimit=0
  Sum : Sum  Inputs=+-  SaturateOnIntegerOverflow=on  InputSameDT=on  OutDataTypeStr=Inherit: Same as first input
  p_A : Outport
  wires:
  Sum/1 -> Product/1
  " dV/dt"/1 -> Sum/2
  Q_in/1 -> Sum/1
  " B"/1 -> Product/3
  " V_A"/1 -> Product/2
  Saturation/1 -> p_A/1
  Integrator/1 -> Saturation/1
  Product/1 -> Integrator/1

== system projectmodel/Hoses/Pipe B ==
  B : Inport
  " dV/dt" : Inport  Port=2
  V_B : Inport  Port=3
  " Q_in" : Inport  Port=4
  Integrator : Integrator  InitialCondition=pinitial  AbsoluteTolerance=10
  Product : Product  Inputs=*/*  SaturateOnIntegerOverflow=on  InputSameDT=on  OutDataTypeStr=Inherit: Same as first input
  Saturation : Saturate  UpperLimit=inf  LowerLimit=0
  Sum : Sum  Inputs=+-  SaturateOnIntegerOverflow=on  InputSameDT=on  OutDataTypeStr=Inherit: Same as first input
  p_B : Outport
  wires:
  Product/1 -> Integrator/1
  Integrator/1 -> Saturation/1
  Saturation/1 -> p_B/1
  Sum/1 -> Product/1
  B/1 -> Product/3
  " Q_in"/1 -> Sum/1
  " dV/dt"/1 -> Sum/2
  V_B/1 -> Product/2

== system projectmodel/Mechanism/Cylinder kinematics ==
  Cyl_A_pos : Inport
  Cyl_A_vel : Inport  Port=2
  Cyl_B_pos : Inport  Port=3
  Cyl_B_vel : Inport  Port=4
  joint_pos : Inport  Port=5
  F_in : Inport  Port=6
  Add : Sum  Inputs=+-
  Cylinder length & velocity : Subsystem
  Length of the cylinder body : Constant  Value=Cyl.x_min
  T_hat = r_hat x F_hat : Subsystem
  Tz : Outport
  x : Outport  Port=2
  v : Outport  Port=3
  wires:
  Length of the cylinder body/1 -> Add/2
  Cylinder length & velocity/1(scalar x) -> Add/1
  Cyl_B_pos/1 -> T_hat = r_hat x F_hat/3(cylB_pos), Cylinder length & velocity/3(C2 pos)
  Cyl_A_vel/1 -> Cylinder length & velocity/2(C1 vel)
  Add/1 -> x/1
  Cylinder length & velocity/2(scalar v) -> v/1
  Cyl_A_pos/1 -> T_hat = r_hat x F_hat/4(cylA_pos), Cylinder length & velocity/1(C1 pos)
  joint_pos/1 -> T_hat = r_hat x F_hat/2(joint_pos)
  Cyl_B_vel/1 -> Cylinder length & velocity/4(C2 vel)
  F_in/1 -> T_hat = r_hat x F_hat/1(F)
  T_hat = r_hat x F_hat/1(Tz) -> Tz/1

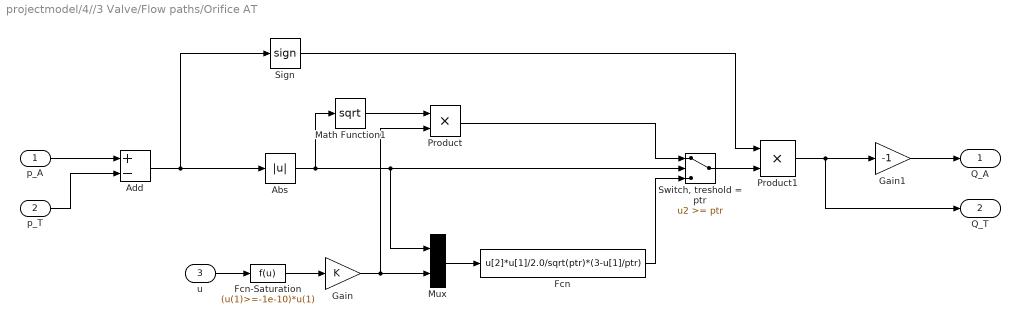
== system projectmodel/4//3 Valve/Flow paths/Orifice AT ==
  p_A : Inport
  p_T : Inport  Port=2
  u : Inport  Port=3
  Abs : Abs  ZeroCross=off  SaturateOnIntegerOverflow=on
  Add : Sum  Inputs=+-
  Fcn : Fcn  Expr=u[2]*u[1]/2.0/sqrt(ptr)*(3-u[1]/ptr)
  Fcn-Saturation : Fcn  Expr=(u(1)>=-1e-10)*u(1)
  Gain : Gain  Gain=K  SaturateOnIntegerOverflow=on  OutDataTypeStr=Inherit: Same as input  ParamDataTypeStr=Inherit: Same as input
  Gain1 : Gain  Gain=-1  SaturateOnIntegerOverflow=on  OutDataTypeStr=Inherit: Same as input  ParamDataTypeStr=Inherit: Same as input
  Math Function1 : Math  Operator=sqrt  SaturateOnIntegerOverflow=on
  Mux : Mux  Inputs=2
  Product : Product  SaturateOnIntegerOverflow=on  InputSameDT=on  OutDataTypeStr=Inherit: Same as first input
  Product1 : Product  SaturateOnIntegerOverflow=on  InputSameDT=on  OutDataTypeStr=Inherit: Same as first input
  Sign : Signum  ZeroCross=off
  "Switch, treshold = ptr" : Switch  Threshold=ptr  ZeroCross=off  SaturateOnIntegerOverflow=on
  Q_A : Outport  InitialOutput=0
  Q_T : Outport  Port=2  InitialOutput=0
  wires:
  u/1 -> Fcn-Saturation/1
  Fcn/1 -> "Switch, treshold = ptr"/3
  Mux/1 -> Fcn/1
  Product/1 -> "Switch, treshold = ptr"/1
  Math Function1/1 -> Product/1
  Abs/1 -> "Switch, treshold = ptr"/2, Mux/1, Math Function1/1
  Fcn-Saturation/1 -> Gain/1
  Gain/1 -> Product/2, Mux/2
  "Switch, treshold = ptr"/1 -> Product1/2
  Sign/1 -> Product1/1
  p_A/1 -> Add/1
  p_T/1 -> Add/2
  Add/1 -> Abs/1, Sign/1
  Product1/1 -> Q_T/1, Gain1/1
  Gain1/1 -> Q_A/1

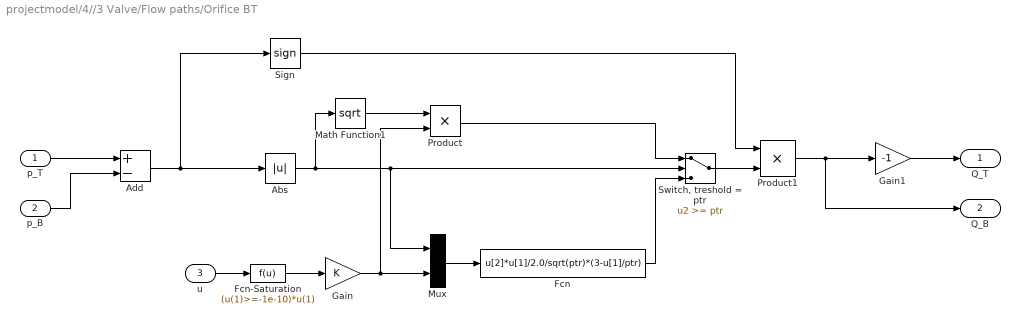
== system projectmodel/4//3 Valve/Flow paths/Orifice BT ==
  p_T : Inport
  p_B : Inport  Port=2
  u : Inport  Port=3
  Abs : Abs  ZeroCross=off  SaturateOnIntegerOverflow=on
  Add : Sum  Inputs=+-
  Fcn : Fcn  Expr=u[2]*u[1]/2.0/sqrt(ptr)*(3-u[1]/ptr)
  Fcn-Saturation : Fcn  Expr=(u(1)>=-1e-10)*u(1)
  Gain : Gain  Gain=K  SaturateOnIntegerOverflow=on  OutDataTypeStr=Inherit: Same as input  ParamDataTypeStr=Inherit: Same as input
  Gain1 : Gain  Gain=-1  SaturateOnIntegerOverflow=on  OutDataTypeStr=Inherit: Same as input  ParamDataTypeStr=Inherit: Same as input
  Math Function1 : Math  Operator=sqrt  SaturateOnIntegerOverflow=on
  Mux : Mux  Inputs=2
  Product : Product  SaturateOnIntegerOverflow=on  InputSameDT=on  OutDataTypeStr=Inherit: Same as first input
  Product1 : Product  SaturateOnIntegerOverflow=on  InputSameDT=on  OutDataTypeStr=Inherit: Same as first input
  Sign : Signum  ZeroCross=off
  "Switch, treshold = ptr" : Switch  Threshold=ptr  ZeroCross=off  SaturateOnIntegerOverflow=on
  Q_T : Outport  InitialOutput=0
  Q_B : Outport  Port=2  InitialOutput=0
  wires:
  Gain1/1 -> Q_T/1
  Product1/1 -> Gain1/1, Q_B/1
  Add/1 -> Sign/1, Abs/1
  p_B/1 -> Add/2
  p_T/1 -> Add/1
  Sign/1 -> Product1/1
  "Switch, treshold = ptr"/1 -> Product1/2
  Gain/1 -> Mux/2, Product/2
  Fcn-Saturation/1 -> Gain/1
  Abs/1 -> Math Function1/1, Mux/1, "Switch, treshold = ptr"/2
  Math Function1/1 -> Product/1
  Product/1 -> "Switch, treshold = ptr"/1
  Mux/1 -> Fcn/1
  Fcn/1 -> "Switch, treshold = ptr"/3
  u/1 -> Fcn-Saturation/1

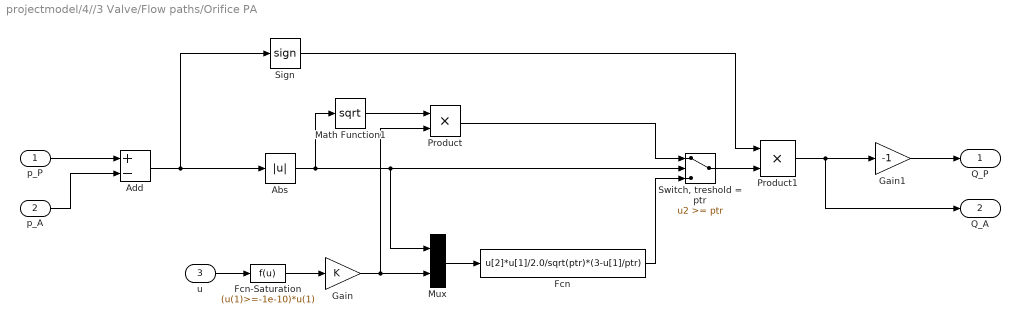
== system projectmodel/4//3 Valve/Flow paths/Orifice PA ==
  p_P : Inport
  p_A : Inport  Port=2
  u : Inport  Port=3
  Abs : Abs  ZeroCross=off  SaturateOnIntegerOverflow=on
  Add : Sum  Inputs=+-
  Fcn : Fcn  Expr=u[2]*u[1]/2.0/sqrt(ptr)*(3-u[1]/ptr)
  Fcn-Saturation : Fcn  Expr=(u(1)>=-1e-10)*u(1)
  Gain : Gain  Gain=K  SaturateOnIntegerOverflow=on  OutDataTypeStr=Inherit: Same as input  ParamDataTypeStr=Inherit: Same as input
  Gain1 : Gain  Gain=-1  SaturateOnIntegerOverflow=on  OutDataTypeStr=Inherit: Same as input  ParamDataTypeStr=Inherit: Same as input
  Math Function1 : Math  Operator=sqrt  SaturateOnIntegerOverflow=on
  Mux : Mux  Inputs=2
  Product : Product  SaturateOnIntegerOverflow=on  InputSameDT=on  OutDataTypeStr=Inherit: Same as first input
  Product1 : Product  SaturateOnIntegerOverflow=on  InputSameDT=on  OutDataTypeStr=Inherit: Same as first input
  Sign : Signum  ZeroCross=off
  "Switch, treshold = ptr" : Switch  Threshold=ptr  ZeroCross=off  SaturateOnIntegerOverflow=on
  Q_P : Outport  InitialOutput=0
  Q_A : Outport  Port=2  InitialOutput=0
  wires:
  u/1 -> Fcn-Saturation/1
  Fcn/1 -> "Switch, treshold = ptr"/3
  Mux/1 -> Fcn/1
  Product/1 -> "Switch, treshold = ptr"/1
  Math Function1/1 -> Product/1
  Abs/1 -> "Switch, treshold = ptr"/2, Mux/1, Math Function1/1
  Fcn-Saturation/1 -> Gain/1
  Gain/1 -> Product/2, Mux/2
  "Switch, treshold = ptr"/1 -> Product1/2
  Sign/1 -> Product1/1
  p_P/1 -> Add/1
  p_A/1 -> Add/2
  Add/1 -> Abs/1, Sign/1
  Product1/1 -> Q_A/1, Gain1/1
  Gain1/1 -> Q_P/1

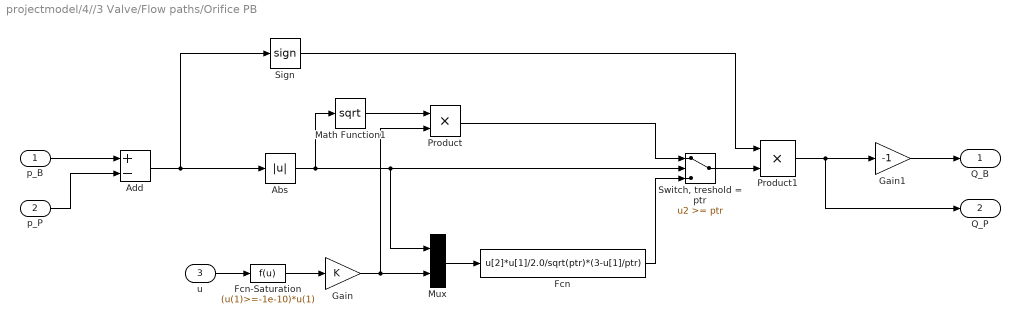
== system projectmodel/4//3 Valve/Flow paths/Orifice PB ==
  p_B : Inport
  p_P : Inport  Port=2
  u : Inport  Port=3
  Abs : Abs  ZeroCross=off  SaturateOnIntegerOverflow=on
  Add : Sum  Inputs=+-
  Fcn : Fcn  Expr=u[2]*u[1]/2.0/sqrt(ptr)*(3-u[1]/ptr)
  Fcn-Saturation : Fcn  Expr=(u(1)>=-1e-10)*u(1)
  Gain : Gain  Gain=K  SaturateOnIntegerOverflow=on  OutDataTypeStr=Inherit: Same as input  ParamDataTypeStr=Inherit: Same as input
  Gain1 : Gain  Gain=-1  SaturateOnIntegerOverflow=on  OutDataTypeStr=Inherit: Same as input  ParamDataTypeStr=Inherit: Same as input
  Math Function1 : Math  Operator=sqrt  SaturateOnIntegerOverflow=on
  Mux : Mux  Inputs=2
  Product : Product  SaturateOnIntegerOverflow=on  InputSameDT=on  OutDataTypeStr=Inherit: Same as first input
  Product1 : Product  SaturateOnIntegerOverflow=on  InputSameDT=on  OutDataTypeStr=Inherit: Same as first input
  Sign : Signum  ZeroCross=off
  "Switch, treshold = ptr" : Switch  Threshold=ptr  ZeroCross=off  SaturateOnIntegerOverflow=on
  Q_B : Outport  InitialOutput=0
  Q_P : Outport  Port=2  InitialOutput=0
  wires:
  Gain1/1 -> Q_B/1
  Product1/1 -> Gain1/1, Q_P/1
  Add/1 -> Sign/1, Abs/1
  p_P/1 -> Add/2
  p_B/1 -> Add/1
  Sign/1 -> Product1/1
  "Switch, treshold = ptr"/1 -> Product1/2
  Gain/1 -> Mux/2, Product/2
  Fcn-Saturation/1 -> Gain/1
  Abs/1 -> Math Function1/1, Mux/1, "Switch, treshold = ptr"/2
  Math Function1/1 -> Product/1
  Product/1 -> "Switch, treshold = ptr"/1
  Mux/1 -> Fcn/1
  Fcn/1 -> "Switch, treshold = ptr"/3
  u/1 -> Fcn-Saturation/1

== system projectmodel/Mechanism/Cylinder kinematics/Cylinder length & velocity ==
  note: v
  note: x
  note: v_hat
  note: x_hat
  C1 pos : Inport
  C1 vel : Inport  Port=2
  C2 pos : Inport  Port=3
  C2 vel : Inport  Port=4
  Add : Sum  Inputs=+-
  Add1 : Sum  Inputs=+-
  Divide : Product  Inputs=/*
  Dot Product : DotProduct  InputSameDT=on  OutDataTypeStr=Inherit: Inherit via internal rule
  norm (length of a vector) : Fcn  Expr=sqrt(u(1)^2+u(2)^2+u(3)^2)
  scalar x : Outport
  scalar v : Outport  Port=2
  wires:
  norm (length of a vector)/1 -> scalar x/1, Divide/1
  C1 vel/1 -> Add1/1
  C2 pos/1 -> Add/2
  C1 pos/1 -> Add/1
  C2 vel/1 -> Add1/2
  Add1/1 -> Dot Product/2
  Divide/1 -> Dot Product/1
  Dot Product/1 -> scalar v/1
  Add/1 -> Divide/2, norm (length of a vector)/1

== system projectmodel/Mechanism/Cylinder kinematics/T_hat = r_hat x F_hat ==
  note: T_hat
  F : Inport
  joint_pos : Inport  Port=2
  cylB_pos : Inport  Port=3
  cylA_pos : Inport  Port=4
  Add : Sum  Inputs=-+
  Add1 : Sum  Inputs=+-
  Cross Product : vrlib/Utilities/Cross Product
  Demux : Demux  Outputs=3
  Normalize Vector (unity vector of xhat)) : vrlib/Utilities/Normalize Vector  maxzero=0
  Product : Product
  Terminator : Terminator
  Terminator1 : Terminator
  Tz : Outport
  wires:
  cylA_pos/1 -> Add1/2
  Demux/1 -> Terminator/1
  Normalize Vector (unity vector of xhat))/1 -> Product/2
  cylB_pos/1 -> Add1/1, Add/2
  Demux/2 -> Terminator1/1
  F/1 -> Product/1
  Cross Product/1 -> Demux/1
  joint_pos/1 -> Add/1
  Add1/1 -> Normalize Vector (unity vector of xhat))/1
  Add/1 -> Cross Product/1
  Product/1 -> Cross Product/2
  Demux/3 -> Tz/1
